simulink model "Feeder_1"  (Simulink 8.8)
settings: Solver=ode4  StartTime=0.0  StopTime=inf  FixedStep=Ts  RelTol=1e-3  EnableMultiTasking=on
PreLoadFcn:
  | Ts=125e-6;Core_Num = 0; np=1; nq=1; Vmin=.9;
PostLoadFcn:
  | Ts=125e-6;Core_Num = 0; np=1; nq=1; Vmin=.9;
InitFcn:
  | Ts=125e-6;Core_Num = 0; np=1; nq=1; Vmin=.9;
undefined symbols (not defined in the file or in its folder): another_event_name, DiscIntNeverNeededParam, I, j, Left, my_event_name, Right, type, V, X
libraries: powerlib x316, powerlib_meascontrol x227, simulink_extras x78, simulink x25, rtio_generic_c37_118 x22, ssn_lib x9, rtlab x6, powerlib_extras x3, artemis x1, rtio_opalrt_ml605ex1 x1, rtio_spectracom x1, rtio_generic_ethernet x1
(part 12 of 14)

== system Feeder_1/SM_NG/Single-Phase Dynamic Load48/model/PLL/adaptive filter ==
  u : Inport
  freq (Hz) : Inport  Port=2
  Gain : Gain  Gain=2*pi*2*0.707*2
  Gain1 : Gain  Gain=2*pi*2
  Product1 : Product  Inputs=***  RndMeth=Zero
  Product2 : Product  Inputs=**  RndMeth=Zero
  Product3 : Product  Inputs=***  RndMeth=Zero
  Sum1 : Sum  Inputs=+--  SaturateOnIntegerOverflow=on  InputSameDT=on  OutDataTypeStr=Inherit: Same as first input
  integrator1 : Integrator
  integrator2 : Integrator
  y : Outport
  wires:
  Product1/1 -> Sum1/2
  u/1 -> Product3/3
  freq (Hz)/1 -> Gain/1, Gain1/1
  Gain1/1 -> Product1/3, Product1/2, Product3/2, Product3/1
  Product3/1 -> Sum1/1
  integrator1/1 -> Product1/1, y/1
  Gain/1 -> Product2/2
  Product2/1 -> Sum1/3
  Sum1/1 -> integrator2/1
  integrator2/1 -> Product2/1, integrator1/1

== system Feeder_1/SM_NG/Single-Phase Dynamic Load48/model/PLL/adaptive mean ==
  u : Inport
  freq (Hz) : Inport  Port=2
  Fcn : Fcn  Expr=u(1)+1e-6
  Math Function : Math  Operator=reciprocal  SaturateOnIntegerOverflow=on
  Product1 : Product  Inputs=**  RndMeth=Zero
  Sum : Sum  Inputs=+-  SaturateOnIntegerOverflow=on  InputSameDT=on  OutDataTypeStr=Inherit: Same as first input
  Variable Transport Delay : VariableTransportDelay  MaximumDelay=1/40  MaximumPoints=4096
  integrator : Integrator
  y : Outport
  wires:
  Product1/1 -> y/1
  u/1 -> integrator/1
  Sum/1 -> Product1/1
  integrator/1 -> Variable Transport Delay/1, Sum/1
  Variable Transport Delay/1 -> Sum/2
  Math Function/1 -> Variable Transport Delay/2
  freq (Hz)/1 -> Fcn/1
  Fcn/1 -> Math Function/1, Product1/2

== system Feeder_1/SM_NG/Single-Phase Dynamic Load49/model/PLL/adaptive filter ==
  u : Inport
  freq (Hz) : Inport  Port=2
  Gain : Gain  Gain=2*pi*2*0.707*2
  Gain1 : Gain  Gain=2*pi*2
  Product1 : Product  Inputs=***  RndMeth=Zero
  Product2 : Product  Inputs=**  RndMeth=Zero
  Product3 : Product  Inputs=***  RndMeth=Zero
  Sum1 : Sum  Inputs=+--  SaturateOnIntegerOverflow=on  InputSameDT=on  OutDataTypeStr=Inherit: Same as first input
  integrator1 : Integrator
  integrator2 : Integrator
  y : Outport
  wires:
  Product1/1 -> Sum1/2
  u/1 -> Product3/3
  freq (Hz)/1 -> Gain/1, Gain1/1
  Gain1/1 -> Product1/3, Product1/2, Product3/2, Product3/1
  Product3/1 -> Sum1/1
  integrator1/1 -> Product1/1, y/1
  Gain/1 -> Product2/2
  Product2/1 -> Sum1/3
  Sum1/1 -> integrator2/1
  integrator2/1 -> Product2/1, integrator1/1

== system Feeder_1/SM_NG/Single-Phase Dynamic Load49/model/PLL/adaptive mean ==
  u : Inport
  freq (Hz) : Inport  Port=2
  Fcn : Fcn  Expr=u(1)+1e-6
  Math Function : Math  Operator=reciprocal  SaturateOnIntegerOverflow=on
  Product1 : Product  Inputs=**  RndMeth=Zero
  Sum : Sum  Inputs=+-  SaturateOnIntegerOverflow=on  InputSameDT=on  OutDataTypeStr=Inherit: Same as first input
  Variable Transport Delay : VariableTransportDelay  MaximumDelay=1/40  MaximumPoints=4096
  integrator : Integrator
  y : Outport
  wires:
  Product1/1 -> y/1
  u/1 -> integrator/1
  Sum/1 -> Product1/1
  integrator/1 -> Variable Transport Delay/1, Sum/1
  Variable Transport Delay/1 -> Sum/2
  Math Function/1 -> Variable Transport Delay/2
  freq (Hz)/1 -> Fcn/1
  Fcn/1 -> Math Function/1, Product1/2

== system Feeder_1/SM_NG/Single-Phase Dynamic Load50/model/PLL/adaptive filter ==
  u : Inport
  freq (Hz) : Inport  Port=2
  Gain : Gain  Gain=2*pi*2*0.707*2
  Gain1 : Gain  Gain=2*pi*2
  Product1 : Product  Inputs=***  RndMeth=Zero
  Product2 : Product  Inputs=**  RndMeth=Zero
  Product3 : Product  Inputs=***  RndMeth=Zero
  Sum1 : Sum  Inputs=+--  SaturateOnIntegerOverflow=on  InputSameDT=on  OutDataTypeStr=Inherit: Same as first input
  integrator1 : Integrator
  integrator2 : Integrator
  y : Outport
  wires:
  Product1/1 -> Sum1/2
  u/1 -> Product3/3
  freq (Hz)/1 -> Gain/1, Gain1/1
  Gain1/1 -> Product1/3, Product1/2, Product3/2, Product3/1
  Product3/1 -> Sum1/1
  integrator1/1 -> Product1/1, y/1
  Gain/1 -> Product2/2
  Product2/1 -> Sum1/3
  Sum1/1 -> integrator2/1
  integrator2/1 -> Product2/1, integrator1/1

== system Feeder_1/SM_NG/Single-Phase Dynamic Load50/model/PLL/adaptive mean ==
  u : Inport
  freq (Hz) : Inport  Port=2
  Fcn : Fcn  Expr=u(1)+1e-6
  Math Function : Math  Operator=reciprocal  SaturateOnIntegerOverflow=on
  Product1 : Product  Inputs=**  RndMeth=Zero
  Sum : Sum  Inputs=+-  SaturateOnIntegerOverflow=on  InputSameDT=on  OutDataTypeStr=Inherit: Same as first input
  Variable Transport Delay : VariableTransportDelay  MaximumDelay=1/40  MaximumPoints=4096
  integrator : Integrator
  y : Outport
  wires:
  Product1/1 -> y/1
  u/1 -> integrator/1
  Sum/1 -> Product1/1
  integrator/1 -> Variable Transport Delay/1, Sum/1
  Variable Transport Delay/1 -> Sum/2
  Math Function/1 -> Variable Transport Delay/2
  freq (Hz)/1 -> Fcn/1
  Fcn/1 -> Math Function/1, Product1/2

== system Feeder_1/SM_NG/Single-Phase Dynamic Load51/model/PLL/adaptive filter ==
  u : Inport
  freq (Hz) : Inport  Port=2
  Gain : Gain  Gain=2*pi*2*0.707*2
  Gain1 : Gain  Gain=2*pi*2
  Product1 : Product  Inputs=***  RndMeth=Zero
  Product2 : Product  Inputs=**  RndMeth=Zero
  Product3 : Product  Inputs=***  RndMeth=Zero
  Sum1 : Sum  Inputs=+--  SaturateOnIntegerOverflow=on  InputSameDT=on  OutDataTypeStr=Inherit: Same as first input
  integrator1 : Integrator
  integrator2 : Integrator
  y : Outport
  wires:
  Product1/1 -> Sum1/2
  u/1 -> Product3/3
  freq (Hz)/1 -> Gain/1, Gain1/1
  Gain1/1 -> Product1/3, Product1/2, Product3/2, Product3/1
  Product3/1 -> Sum1/1
  integrator1/1 -> Product1/1, y/1
  Gain/1 -> Product2/2
  Product2/1 -> Sum1/3
  Sum1/1 -> integrator2/1
  integrator2/1 -> Product2/1, integrator1/1

== system Feeder_1/SM_NG/Single-Phase Dynamic Load51/model/PLL/adaptive mean ==
  u : Inport
  freq (Hz) : Inport  Port=2
  Fcn : Fcn  Expr=u(1)+1e-6
  Math Function : Math  Operator=reciprocal  SaturateOnIntegerOverflow=on
  Product1 : Product  Inputs=**  RndMeth=Zero
  Sum : Sum  Inputs=+-  SaturateOnIntegerOverflow=on  InputSameDT=on  OutDataTypeStr=Inherit: Same as first input
  Variable Transport Delay : VariableTransportDelay  MaximumDelay=1/40  MaximumPoints=4096
  integrator : Integrator
  y : Outport
  wires:
  Product1/1 -> y/1
  u/1 -> integrator/1
  Sum/1 -> Product1/1
  integrator/1 -> Variable Transport Delay/1, Sum/1
  Variable Transport Delay/1 -> Sum/2
  Math Function/1 -> Variable Transport Delay/2
  freq (Hz)/1 -> Fcn/1
  Fcn/1 -> Math Function/1, Product1/2

== system Feeder_1/SM_NG/Single-Phase Dynamic Load52/model/PLL/adaptive filter ==
  u : Inport
  freq (Hz) : Inport  Port=2
  Gain : Gain  Gain=2*pi*2*0.707*2
  Gain1 : Gain  Gain=2*pi*2
  Product1 : Product  Inputs=***  RndMeth=Zero
  Product2 : Product  Inputs=**  RndMeth=Zero
  Product3 : Product  Inputs=***  RndMeth=Zero
  Sum1 : Sum  Inputs=+--  SaturateOnIntegerOverflow=on  InputSameDT=on  OutDataTypeStr=Inherit: Same as first input
  integrator1 : Integrator
  integrator2 : Integrator
  y : Outport
  wires:
  Product1/1 -> Sum1/2
  u/1 -> Product3/3
  freq (Hz)/1 -> Gain/1, Gain1/1
  Gain1/1 -> Product1/3, Product1/2, Product3/2, Product3/1
  Product3/1 -> Sum1/1
  integrator1/1 -> Product1/1, y/1
  Gain/1 -> Product2/2
  Product2/1 -> Sum1/3
  Sum1/1 -> integrator2/1
  integrator2/1 -> Product2/1, integrator1/1

== system Feeder_1/SM_NG/Single-Phase Dynamic Load52/model/PLL/adaptive mean ==
  u : Inport
  freq (Hz) : Inport  Port=2
  Fcn : Fcn  Expr=u(1)+1e-6
  Math Function : Math  Operator=reciprocal  SaturateOnIntegerOverflow=on
  Product1 : Product  Inputs=**  RndMeth=Zero
  Sum : Sum  Inputs=+-  SaturateOnIntegerOverflow=on  InputSameDT=on  OutDataTypeStr=Inherit: Same as first input
  Variable Transport Delay : VariableTransportDelay  MaximumDelay=1/40  MaximumPoints=4096
  integrator : Integrator
  y : Outport
  wires:
  Product1/1 -> y/1
  u/1 -> integrator/1
  Sum/1 -> Product1/1
  integrator/1 -> Variable Transport Delay/1, Sum/1
  Variable Transport Delay/1 -> Sum/2
  Math Function/1 -> Variable Transport Delay/2
  freq (Hz)/1 -> Fcn/1
  Fcn/1 -> Math Function/1, Product1/2

== system Feeder_1/SM_NG/Single-Phase Dynamic Load53/model/PLL/adaptive filter ==
  u : Inport
  freq (Hz) : Inport  Port=2
  Gain : Gain  Gain=2*pi*2*0.707*2
  Gain1 : Gain  Gain=2*pi*2
  Product1 : Product  Inputs=***  RndMeth=Zero
  Product2 : Product  Inputs=**  RndMeth=Zero
  Product3 : Product  Inputs=***  RndMeth=Zero
  Sum1 : Sum  Inputs=+--  SaturateOnIntegerOverflow=on  InputSameDT=on  OutDataTypeStr=Inherit: Same as first input
  integrator1 : Integrator
  integrator2 : Integrator
  y : Outport
  wires:
  Product1/1 -> Sum1/2
  u/1 -> Product3/3
  freq (Hz)/1 -> Gain/1, Gain1/1
  Gain1/1 -> Product1/3, Product1/2, Product3/2, Product3/1
  Product3/1 -> Sum1/1
  integrator1/1 -> Product1/1, y/1
  Gain/1 -> Product2/2
  Product2/1 -> Sum1/3
  Sum1/1 -> integrator2/1
  integrator2/1 -> Product2/1, integrator1/1

== system Feeder_1/SM_NG/Single-Phase Dynamic Load53/model/PLL/adaptive mean ==
  u : Inport
  freq (Hz) : Inport  Port=2
  Fcn : Fcn  Expr=u(1)+1e-6
  Math Function : Math  Operator=reciprocal  SaturateOnIntegerOverflow=on
  Product1 : Product  Inputs=**  RndMeth=Zero
  Sum : Sum  Inputs=+-  SaturateOnIntegerOverflow=on  InputSameDT=on  OutDataTypeStr=Inherit: Same as first input
  Variable Transport Delay : VariableTransportDelay  MaximumDelay=1/40  MaximumPoints=4096
  integrator : Integrator
  y : Outport
  wires:
  Product1/1 -> y/1
  u/1 -> integrator/1
  Sum/1 -> Product1/1
  integrator/1 -> Variable Transport Delay/1, Sum/1
  Variable Transport Delay/1 -> Sum/2
  Math Function/1 -> Variable Transport Delay/2
  freq (Hz)/1 -> Fcn/1
  Fcn/1 -> Math Function/1, Product1/2

== system Feeder_1/SM_NG/Single-Phase Dynamic Load54/model/PLL/adaptive filter ==
  u : Inport
  freq (Hz) : Inport  Port=2
  Gain : Gain  Gain=2*pi*2*0.707*2
  Gain1 : Gain  Gain=2*pi*2
  Product1 : Product  Inputs=***  RndMeth=Zero
  Product2 : Product  Inputs=**  RndMeth=Zero
  Product3 : Product  Inputs=***  RndMeth=Zero
  Sum1 : Sum  Inputs=+--  SaturateOnIntegerOverflow=on  InputSameDT=on  OutDataTypeStr=Inherit: Same as first input
  integrator1 : Integrator
  integrator2 : Integrator
  y : Outport
  wires:
  Product1/1 -> Sum1/2
  u/1 -> Product3/3
  freq (Hz)/1 -> Gain/1, Gain1/1
  Gain1/1 -> Product1/3, Product1/2, Product3/2, Product3/1
  Product3/1 -> Sum1/1
  integrator1/1 -> Product1/1, y/1
  Gain/1 -> Product2/2
  Product2/1 -> Sum1/3
  Sum1/1 -> integrator2/1
  integrator2/1 -> Product2/1, integrator1/1

== system Feeder_1/SM_NG/Single-Phase Dynamic Load54/model/PLL/adaptive mean ==
  u : Inport
  freq (Hz) : Inport  Port=2
  Fcn : Fcn  Expr=u(1)+1e-6
  Math Function : Math  Operator=reciprocal  SaturateOnIntegerOverflow=on
  Product1 : Product  Inputs=**  RndMeth=Zero
  Sum : Sum  Inputs=+-  SaturateOnIntegerOverflow=on  InputSameDT=on  OutDataTypeStr=Inherit: Same as first input
  Variable Transport Delay : VariableTransportDelay  MaximumDelay=1/40  MaximumPoints=4096
  integrator : Integrator
  y : Outport
  wires:
  Product1/1 -> y/1
  u/1 -> integrator/1
  Sum/1 -> Product1/1
  integrator/1 -> Variable Transport Delay/1, Sum/1
  Variable Transport Delay/1 -> Sum/2
  Math Function/1 -> Variable Transport Delay/2
  freq (Hz)/1 -> Fcn/1
  Fcn/1 -> Math Function/1, Product1/2

== system Feeder_1/SM_NG/Single-Phase Dynamic Load55/model/PLL/adaptive filter ==
  u : Inport
  freq (Hz) : Inport  Port=2
  Gain : Gain  Gain=2*pi*2*0.707*2
  Gain1 : Gain  Gain=2*pi*2
  Product1 : Product  Inputs=***  RndMeth=Zero
  Product2 : Product  Inputs=**  RndMeth=Zero
  Product3 : Product  Inputs=***  RndMeth=Zero
  Sum1 : Sum  Inputs=+--  SaturateOnIntegerOverflow=on  InputSameDT=on  OutDataTypeStr=Inherit: Same as first input
  integrator1 : Integrator
  integrator2 : Integrator
  y : Outport
  wires:
  Product1/1 -> Sum1/2
  u/1 -> Product3/3
  freq (Hz)/1 -> Gain/1, Gain1/1
  Gain1/1 -> Product1/3, Product1/2, Product3/2, Product3/1
  Product3/1 -> Sum1/1
  integrator1/1 -> Product1/1, y/1
  Gain/1 -> Product2/2
  Product2/1 -> Sum1/3
  Sum1/1 -> integrator2/1
  integrator2/1 -> Product2/1, integrator1/1

== system Feeder_1/SM_NG/Single-Phase Dynamic Load55/model/PLL/adaptive mean ==
  u : Inport
  freq (Hz) : Inport  Port=2
  Fcn : Fcn  Expr=u(1)+1e-6
  Math Function : Math  Operator=reciprocal  SaturateOnIntegerOverflow=on
  Product1 : Product  Inputs=**  RndMeth=Zero
  Sum : Sum  Inputs=+-  SaturateOnIntegerOverflow=on  InputSameDT=on  OutDataTypeStr=Inherit: Same as first input
  Variable Transport Delay : VariableTransportDelay  MaximumDelay=1/40  MaximumPoints=4096
  integrator : Integrator
  y : Outport
  wires:
  Product1/1 -> y/1
  u/1 -> integrator/1
  Sum/1 -> Product1/1
  integrator/1 -> Variable Transport Delay/1, Sum/1
  Variable Transport Delay/1 -> Sum/2
  Math Function/1 -> Variable Transport Delay/2
  freq (Hz)/1 -> Fcn/1
  Fcn/1 -> Math Function/1, Product1/2

== system Feeder_1/SM_NG/Single-Phase Dynamic Load56/model/PLL/adaptive filter ==
  u : Inport
  freq (Hz) : Inport  Port=2
  Gain : Gain  Gain=2*pi*2*0.707*2
  Gain1 : Gain  Gain=2*pi*2
  Product1 : Product  Inputs=***  RndMeth=Zero
  Product2 : Product  Inputs=**  RndMeth=Zero
  Product3 : Product  Inputs=***  RndMeth=Zero
  Sum1 : Sum  Inputs=+--  SaturateOnIntegerOverflow=on  InputSameDT=on  OutDataTypeStr=Inherit: Same as first input
  integrator1 : Integrator
  integrator2 : Integrator
  y : Outport
  wires:
  Product1/1 -> Sum1/2
  u/1 -> Product3/3
  freq (Hz)/1 -> Gain/1, Gain1/1
  Gain1/1 -> Product1/3, Product1/2, Product3/2, Product3/1
  Product3/1 -> Sum1/1
  integrator1/1 -> Product1/1, y/1
  Gain/1 -> Product2/2
  Product2/1 -> Sum1/3
  Sum1/1 -> integrator2/1
  integrator2/1 -> Product2/1, integrator1/1

== system Feeder_1/SM_NG/Single-Phase Dynamic Load56/model/PLL/adaptive mean ==
  u : Inport
  freq (Hz) : Inport  Port=2
  Fcn : Fcn  Expr=u(1)+1e-6
  Math Function : Math  Operator=reciprocal  SaturateOnIntegerOverflow=on
  Product1 : Product  Inputs=**  RndMeth=Zero
  Sum : Sum  Inputs=+-  SaturateOnIntegerOverflow=on  InputSameDT=on  OutDataTypeStr=Inherit: Same as first input
  Variable Transport Delay : VariableTransportDelay  MaximumDelay=1/40  MaximumPoints=4096
  integrator : Integrator
  y : Outport
  wires:
  Product1/1 -> y/1
  u/1 -> integrator/1
  Sum/1 -> Product1/1
  integrator/1 -> Variable Transport Delay/1, Sum/1
  Variable Transport Delay/1 -> Sum/2
  Math Function/1 -> Variable Transport Delay/2
  freq (Hz)/1 -> Fcn/1
  Fcn/1 -> Math Function/1, Product1/2

== system Feeder_1/SM_NG/Single-Phase Dynamic Load57/model/PLL/adaptive filter ==
  u : Inport
  freq (Hz) : Inport  Port=2
  Gain : Gain  Gain=2*pi*2*0.707*2
  Gain1 : Gain  Gain=2*pi*2
  Product1 : Product  Inputs=***  RndMeth=Zero
  Product2 : Product  Inputs=**  RndMeth=Zero
  Product3 : Product  Inputs=***  RndMeth=Zero
  Sum1 : Sum  Inputs=+--  SaturateOnIntegerOverflow=on  InputSameDT=on  OutDataTypeStr=Inherit: Same as first input
  integrator1 : Integrator
  integrator2 : Integrator
  y : Outport
  wires:
  Product1/1 -> Sum1/2
  u/1 -> Product3/3
  freq (Hz)/1 -> Gain/1, Gain1/1
  Gain1/1 -> Product1/3, Product1/2, Product3/2, Product3/1
  Product3/1 -> Sum1/1
  integrator1/1 -> Product1/1, y/1
  Gain/1 -> Product2/2
  Product2/1 -> Sum1/3
  Sum1/1 -> integrator2/1
  integrator2/1 -> Product2/1, integrator1/1

== system Feeder_1/SM_NG/Single-Phase Dynamic Load57/model/PLL/adaptive mean ==
  u : Inport
  freq (Hz) : Inport  Port=2
  Fcn : Fcn  Expr=u(1)+1e-6
  Math Function : Math  Operator=reciprocal  SaturateOnIntegerOverflow=on
  Product1 : Product  Inputs=**  RndMeth=Zero
  Sum : Sum  Inputs=+-  SaturateOnIntegerOverflow=on  InputSameDT=on  OutDataTypeStr=Inherit: Same as first input
  Variable Transport Delay : VariableTransportDelay  MaximumDelay=1/40  MaximumPoints=4096
  integrator : Integrator
  y : Outport
  wires:
  Product1/1 -> y/1
  u/1 -> integrator/1
  Sum/1 -> Product1/1
  integrator/1 -> Variable Transport Delay/1, Sum/1
  Variable Transport Delay/1 -> Sum/2
  Math Function/1 -> Variable Transport Delay/2
  freq (Hz)/1 -> Fcn/1
  Fcn/1 -> Math Function/1, Product1/2

== system Feeder_1/SM_NG/Single-Phase Dynamic Load58/model/PLL/adaptive filter ==
  u : Inport
  freq (Hz) : Inport  Port=2
  Gain : Gain  Gain=2*pi*2*0.707*2
  Gain1 : Gain  Gain=2*pi*2
  Product1 : Product  Inputs=***  RndMeth=Zero
  Product2 : Product  Inputs=**  RndMeth=Zero
  Product3 : Product  Inputs=***  RndMeth=Zero
  Sum1 : Sum  Inputs=+--  SaturateOnIntegerOverflow=on  InputSameDT=on  OutDataTypeStr=Inherit: Same as first input
  integrator1 : Integrator
  integrator2 : Integrator
  y : Outport
  wires:
  Product1/1 -> Sum1/2
  u/1 -> Product3/3
  freq (Hz)/1 -> Gain/1, Gain1/1
  Gain1/1 -> Product1/3, Product1/2, Product3/2, Product3/1
  Product3/1 -> Sum1/1
  integrator1/1 -> Product1/1, y/1
  Gain/1 -> Product2/2
  Product2/1 -> Sum1/3
  Sum1/1 -> integrator2/1
  integrator2/1 -> Product2/1, integrator1/1

== system Feeder_1/SM_NG/Single-Phase Dynamic Load58/model/PLL/adaptive mean ==
  u : Inport
  freq (Hz) : Inport  Port=2
  Fcn : Fcn  Expr=u(1)+1e-6
  Math Function : Math  Operator=reciprocal  SaturateOnIntegerOverflow=on
  Product1 : Product  Inputs=**  RndMeth=Zero
  Sum : Sum  Inputs=+-  SaturateOnIntegerOverflow=on  InputSameDT=on  OutDataTypeStr=Inherit: Same as first input
  Variable Transport Delay : VariableTransportDelay  MaximumDelay=1/40  MaximumPoints=4096
  integrator : Integrator
  y : Outport
  wires:
  Product1/1 -> y/1
  u/1 -> integrator/1
  Sum/1 -> Product1/1
  integrator/1 -> Variable Transport Delay/1, Sum/1
  Variable Transport Delay/1 -> Sum/2
  Math Function/1 -> Variable Transport Delay/2
  freq (Hz)/1 -> Fcn/1
  Fcn/1 -> Math Function/1, Product1/2

== system Feeder_1/SM_NG/Single-Phase Dynamic Load59/model/PLL/adaptive filter ==
  u : Inport
  freq (Hz) : Inport  Port=2
  Gain : Gain  Gain=2*pi*2*0.707*2
  Gain1 : Gain  Gain=2*pi*2
  Product1 : Product  Inputs=***  RndMeth=Zero
  Product2 : Product  Inputs=**  RndMeth=Zero
  Product3 : Product  Inputs=***  RndMeth=Zero
  Sum1 : Sum  Inputs=+--  SaturateOnIntegerOverflow=on  InputSameDT=on  OutDataTypeStr=Inherit: Same as first input
  integrator1 : Integrator
  integrator2 : Integrator
  y : Outport
  wires:
  Product1/1 -> Sum1/2
  u/1 -> Product3/3
  freq (Hz)/1 -> Gain/1, Gain1/1
  Gain1/1 -> Product1/3, Product1/2, Product3/2, Product3/1
  Product3/1 -> Sum1/1
  integrator1/1 -> Product1/1, y/1
  Gain/1 -> Product2/2
  Product2/1 -> Sum1/3
  Sum1/1 -> integrator2/1
  integrator2/1 -> Product2/1, integrator1/1

== system Feeder_1/SM_NG/Single-Phase Dynamic Load59/model/PLL/adaptive mean ==
  u : Inport
  freq (Hz) : Inport  Port=2
  Fcn : Fcn  Expr=u(1)+1e-6
  Math Function : Math  Operator=reciprocal  SaturateOnIntegerOverflow=on
  Product1 : Product  Inputs=**  RndMeth=Zero
  Sum : Sum  Inputs=+-  SaturateOnIntegerOverflow=on  InputSameDT=on  OutDataTypeStr=Inherit: Same as first input
  Variable Transport Delay : VariableTransportDelay  MaximumDelay=1/40  MaximumPoints=4096
  integrator : Integrator
  y : Outport
  wires:
  Product1/1 -> y/1
  u/1 -> integrator/1
  Sum/1 -> Product1/1
  integrator/1 -> Variable Transport Delay/1, Sum/1
  Variable Transport Delay/1 -> Sum/2
  Math Function/1 -> Variable Transport Delay/2
  freq (Hz)/1 -> Fcn/1
  Fcn/1 -> Math Function/1, Product1/2

== system Feeder_1/SM_NG/Single-Phase Dynamic Load60/model/PLL/adaptive filter ==
  u : Inport
  freq (Hz) : Inport  Port=2
  Gain : Gain  Gain=2*pi*2*0.707*2
  Gain1 : Gain  Gain=2*pi*2
  Product1 : Product  Inputs=***  RndMeth=Zero
  Product2 : Product  Inputs=**  RndMeth=Zero
  Product3 : Product  Inputs=***  RndMeth=Zero
  Sum1 : Sum  Inputs=+--  SaturateOnIntegerOverflow=on  InputSameDT=on  OutDataTypeStr=Inherit: Same as first input
  integrator1 : Integrator
  integrator2 : Integrator
  y : Outport
  wires:
  Product1/1 -> Sum1/2
  u/1 -> Product3/3
  freq (Hz)/1 -> Gain/1, Gain1/1
  Gain1/1 -> Product1/3, Product1/2, Product3/2, Product3/1
  Product3/1 -> Sum1/1
  integrator1/1 -> Product1/1, y/1
  Gain/1 -> Product2/2
  Product2/1 -> Sum1/3
  Sum1/1 -> integrator2/1
  integrator2/1 -> Product2/1, integrator1/1

== system Feeder_1/SM_NG/Single-Phase Dynamic Load60/model/PLL/adaptive mean ==
  u : Inport
  freq (Hz) : Inport  Port=2
  Fcn : Fcn  Expr=u(1)+1e-6
  Math Function : Math  Operator=reciprocal  SaturateOnIntegerOverflow=on
  Product1 : Product  Inputs=**  RndMeth=Zero
  Sum : Sum  Inputs=+-  SaturateOnIntegerOverflow=on  InputSameDT=on  OutDataTypeStr=Inherit: Same as first input
  Variable Transport Delay : VariableTransportDelay  MaximumDelay=1/40  MaximumPoints=4096
  integrator : Integrator
  y : Outport
  wires:
  Product1/1 -> y/1
  u/1 -> integrator/1
  Sum/1 -> Product1/1
  integrator/1 -> Variable Transport Delay/1, Sum/1
  Variable Transport Delay/1 -> Sum/2
  Math Function/1 -> Variable Transport Delay/2
  freq (Hz)/1 -> Fcn/1
  Fcn/1 -> Math Function/1, Product1/2

== system Feeder_1/SM_NG/Subsystem/Single-Phase Voltage Regulator1/SSN OLTC xfo v2/DC source_a ==
  I1A_V : powerlib/Electrical Sources/DC Voltage Source  Amplitude=0  Measurements=None
  Conn1 : PMIOPort  Port=1  Side=Left
  Conn2 : PMIOPort  Port=2  Side=Right
  connections:
  Conn1/RConn1 -- I1A_V/LConn1
  Conn2/RConn1 -- I1A_V/RConn1

== system Feeder_1/SM_NG/Subsystem/Single-Phase Voltage Regulator1/SSN OLTC xfo v2/DC source_b ==
  I1B_V : powerlib/Electrical Sources/DC Voltage Source  Amplitude=0  Measurements=None
  Conn3 : PMIOPort  Port=1  Side=Left
  Conn4 : PMIOPort  Port=2  Side=Right
  connections:
  Conn4/RConn1 -- I1B_V/RConn1
  Conn3/RConn1 -- I1B_V/LConn1

== system Feeder_1/SM_NG/Subsystem/Single-Phase Voltage Regulator1/SSN OLTC xfo v2/DC source_c ==
  I1C_V : powerlib/Electrical Sources/DC Voltage Source  Amplitude=0  Measurements=None
  Conn1 : PMIOPort  Port=1  Side=Left
  Conn2 : PMIOPort  Port=2  Side=Right
  connections:
  Conn2/RConn1 -- I1C_V/RConn1
  Conn1/RConn1 -- I1C_V/LConn1

== system Feeder_1/SM_NG/Subsystem/Single-Phase Voltage Regulator1/SSN OLTC xfo v2/DC source_d ==
  I1D_V : powerlib/Electrical Sources/DC Voltage Source  Amplitude=0  Measurements=None
  Conn3 : PMIOPort  Port=1  Side=Left
  Conn4 : PMIOPort  Port=2  Side=Right
  connections:
  Conn3/RConn1 -- I1D_V/LConn1
  Conn4/RConn1 -- I1D_V/RConn1

== system Feeder_1/SM_NG/Subsystem/Single-Phase Voltage Regulator1/SSN OLTC xfo v2/SSS-SM equations ==
  A : Inport
  B : Inport  Port=2
  C : Inport  Port=3
  u : Inport  Port=4
  Flux0 : Inport  Port=5
  Bphic : Inport  Port=6
  be : Inport  Port=7
  Constant : Constant
  Discretize : Subsystem
  Product{1..3,5..6} (5 alike) : Product  Multiplication=Matrix(*)  SaturateOnIntegerOverflow=on  OutDataTypeStr=Inherit: Same as first input
  Sum1 : Sum  Inputs=-+  SaturateOnIntegerOverflow=on
  Sum2 : Sum  Inputs=+++  SaturateOnIntegerOverflow=on
  Sum3 : Sum  SaturateOnIntegerOverflow=on
  mult1 : Product
  u5 : Constant  Value=eye(3,3)
  z-1 : UnitDelay  SampleTime=Ts
  Y : Outport
  Ihist : Outport  Port=2
  x : Outport  Port=3
  wires:
  u5/1 -> Discretize/3(Unity)
  Product2/1 -> Y/1
  A/1 -> Discretize/1(Ac)
  B/1 -> Discretize/2(Bc)
  C/1 -> Product2/1, Product6/1
  Product6/1 -> Ihist/1
  Product5/1 -> Sum3/2, mult1/1
  Product3/1 -> Sum2/1
  Sum3/1 -> Product3/2, x/1  "new_x"
  Sum2/1 -> z-1/1, Product6/2
  Discretize/1(Ad) -> Product3/1
  u/1 -> Product5/2
  z-1/1 -> Sum3/1
  Discretize/2(Bd) -> Product5/1, Product2/2
  Discretize/3(Bdin) -> Product1/1
  Product1/1 -> Sum2/3
  Flux0/1 -> Product1/2
  Bphic/1 -> Discretize/4(Bphic)
  Constant/1 -> Sum1/2
  mult1/1 -> Sum2/2
  Sum1/1 -> mult1/2  "=1 if trapeze           =0 if BE"
  be/1 -> Discretize/5(be), Sum1/1

== system Feeder_1/SM_NG/Subsystem/Single-Phase Voltage Regulator1/SSN OLTC xfo v2/Update Matrix L ==
  k : Inport
  L2 : Inport  Port=2
  Lin : Inport  Port=3
  "L2->(2,2) " : Assignment  NumberOfDimensions=2  IndexOptions=Index vector (dialog),Index vector (dialog)  Indices=[2],[2]  OutputSizes=1,1
  k->(2,3) : Assignment  NumberOfDimensions=2  IndexOptions=Index vector (dialog),Index vector (dialog)  Indices=[2],[3]  OutputSizes=1,1
  L : Outport
  wires:
  "L2->(2,2) "/1 -> L/1
  L2/1 -> "L2->(2,2) "/2
  Lin/1 -> k->(2,3)/1
  k/1 -> k->(2,3)/2
  k->(2,3)/1 -> "L2->(2,2) "/1

== system Feeder_1/SM_NG/Subsystem/Single-Phase Voltage Regulator1/SSN OLTC xfo v2/Update Matrix R ==
  R2 : Inport
  Rin : Inport  Port=2
  k : Inport  Port=3
  Rcore : Inport  Port=4
  Rcore/Lcore : Inport  Port=5
  "-R2->(2,2) " : Assignment  NumberOfDimensions=2  IndexOptions=Index vector (dialog),Index vector (dialog)  Indices=[2],[2]  OutputSizes=1,1
  -Rm/Lm->(3,3) : Assignment  NumberOfDimensions=2  IndexOptions=Index vector (dialog),Index vector (dialog)  Indices=3,3  OutputSizes=1,1
  Gain : Gain  Gain=-1
  Gain1 : Gain  Gain=-1
  Product1 : Product  RndMeth=Zero
  kRm->(3,2) : Assignment  NumberOfDimensions=2  IndexOptions=Index vector (dialog),Index vector (dialog)  Indices=3,2  OutputSizes=1,1
  R : Outport
  wires:
  "-R2->(2,2) "/1 -> kRm->(3,2)/1
  R2/1 -> Gain/1
  Rin/1 -> "-R2->(2,2) "/1
  Gain/1 -> "-R2->(2,2) "/2
  k/1 -> Product1/2
  Product1/1 -> kRm->(3,2)/2
  kRm->(3,2)/1 -> -Rm/Lm->(3,3)/1
  -Rm/Lm->(3,3)/1 -> R/1
  Rcore/1 -> Product1/1
  Gain1/1 -> -Rm/Lm->(3,3)/2
  Rcore/Lcore/1 -> Gain1/1

== system Feeder_1/SM_NG/Subsystem/Single-Phase Voltage Regulator1/SSN OLTC xfo v2/conn_down_c ==
  b2 : PMIOPort  Port=1  Side=Right
  b1 : PMIOPort  Port=2  Side=Left
  connections:
  b1/RConn1 -- b2/RConn1

== system Feeder_1/SM_NG/Subsystem/Single-Phase Voltage Regulator1/SSN OLTC xfo v2/conn_down_d ==
  b2 : PMIOPort  Port=1  Side=Right
  b1 : PMIOPort  Port=2  Side=Left
  connections:
  b1/RConn1 -- b2/RConn1

== system Feeder_1/SM_NG/Subsystem/Single-Phase Voltage Regulator1/SSN OLTC xfo v2/conn_up_c ==
  b2 : PMIOPort  Port=1  Side=Right
  b1 : PMIOPort  Port=2  Side=Left
  connections:
  b1/RConn1 -- b2/RConn1

== system Feeder_1/SM_NG/Subsystem/Single-Phase Voltage Regulator1/SSN OLTC xfo v2/conn_up_d ==
  b2 : PMIOPort  Port=1  Side=Right
  b1 : PMIOPort  Port=2  Side=Left
  connections:
  b1/RConn1 -- b2/RConn1

== system Feeder_1/SM_NG/Subsystem/Single-Phase Voltage Regulator2/SSN OLTC xfo v2/DC source_a ==
  I1A_V : powerlib/Electrical Sources/DC Voltage Source  Amplitude=0  Measurements=None
  Conn1 : PMIOPort  Port=1  Side=Left
  Conn2 : PMIOPort  Port=2  Side=Right
  connections:
  Conn1/RConn1 -- I1A_V/LConn1
  Conn2/RConn1 -- I1A_V/RConn1

== system Feeder_1/SM_NG/Subsystem/Single-Phase Voltage Regulator2/SSN OLTC xfo v2/DC source_b ==
  I1B_V : powerlib/Electrical Sources/DC Voltage Source  Amplitude=0  Measurements=None
  Conn3 : PMIOPort  Port=1  Side=Left
  Conn4 : PMIOPort  Port=2  Side=Right
  connections:
  Conn4/RConn1 -- I1B_V/RConn1
  Conn3/RConn1 -- I1B_V/LConn1

== system Feeder_1/SM_NG/Subsystem/Single-Phase Voltage Regulator2/SSN OLTC xfo v2/DC source_c ==
  I1C_V : powerlib/Electrical Sources/DC Voltage Source  Amplitude=0  Measurements=None
  Conn1 : PMIOPort  Port=1  Side=Left
  Conn2 : PMIOPort  Port=2  Side=Right
  connections:
  Conn2/RConn1 -- I1C_V/RConn1
  Conn1/RConn1 -- I1C_V/LConn1

== system Feeder_1/SM_NG/Subsystem/Single-Phase Voltage Regulator2/SSN OLTC xfo v2/DC source_d ==
  I1D_V : powerlib/Electrical Sources/DC Voltage Source  Amplitude=0  Measurements=None
  Conn3 : PMIOPort  Port=1  Side=Left
  Conn4 : PMIOPort  Port=2  Side=Right
  connections:
  Conn3/RConn1 -- I1D_V/LConn1
  Conn4/RConn1 -- I1D_V/RConn1

== system Feeder_1/SM_NG/Subsystem/Single-Phase Voltage Regulator2/SSN OLTC xfo v2/SSS-SM equations ==
  A : Inport
  B : Inport  Port=2
  C : Inport  Port=3
  u : Inport  Port=4
  Flux0 : Inport  Port=5
  Bphic : Inport  Port=6
  be : Inport  Port=7
  Constant : Constant
  Discretize : Subsystem
  Product{1..3,5..6} (5 alike) : Product  Multiplication=Matrix(*)  SaturateOnIntegerOverflow=on  OutDataTypeStr=Inherit: Same as first input
  Sum1 : Sum  Inputs=-+  SaturateOnIntegerOverflow=on
  Sum2 : Sum  Inputs=+++  SaturateOnIntegerOverflow=on
  Sum3 : Sum  SaturateOnIntegerOverflow=on
  mult1 : Product
  u5 : Constant  Value=eye(3,3)
  z-1 : UnitDelay  SampleTime=Ts
  Y : Outport
  Ihist : Outport  Port=2
  x : Outport  Port=3
  wires:
  u5/1 -> Discretize/3(Unity)
  Product2/1 -> Y/1
  A/1 -> Discretize/1(Ac)
  B/1 -> Discretize/2(Bc)
  C/1 -> Product2/1, Product6/1
  Product6/1 -> Ihist/1
  Product5/1 -> Sum3/2, mult1/1
  Product3/1 -> Sum2/1
  Sum3/1 -> Product3/2, x/1  "new_x"
  Sum2/1 -> z-1/1, Product6/2
  Discretize/1(Ad) -> Product3/1
  u/1 -> Product5/2
  z-1/1 -> Sum3/1
  Discretize/2(Bd) -> Product5/1, Product2/2
  Discretize/3(Bdin) -> Product1/1
  Product1/1 -> Sum2/3
  Flux0/1 -> Product1/2
  Bphic/1 -> Discretize/4(Bphic)
  Constant/1 -> Sum1/2
  mult1/1 -> Sum2/2
  Sum1/1 -> mult1/2  "=1 if trapeze           =0 if BE"
  be/1 -> Discretize/5(be), Sum1/1

== system Feeder_1/SM_NG/Subsystem/Single-Phase Voltage Regulator2/SSN OLTC xfo v2/Update Matrix L ==
  k : Inport
  L2 : Inport  Port=2
  Lin : Inport  Port=3
  "L2->(2,2) " : Assignment  NumberOfDimensions=2  IndexOptions=Index vector (dialog),Index vector (dialog)  Indices=[2],[2]  OutputSizes=1,1
  k->(2,3) : Assignment  NumberOfDimensions=2  IndexOptions=Index vector (dialog),Index vector (dialog)  Indices=[2],[3]  OutputSizes=1,1
  L : Outport
  wires:
  "L2->(2,2) "/1 -> L/1
  L2/1 -> "L2->(2,2) "/2
  Lin/1 -> k->(2,3)/1
  k/1 -> k->(2,3)/2
  k->(2,3)/1 -> "L2->(2,2) "/1

== system Feeder_1/SM_NG/Subsystem/Single-Phase Voltage Regulator2/SSN OLTC xfo v2/Update Matrix R ==
  R2 : Inport
  Rin : Inport  Port=2
  k : Inport  Port=3
  Rcore : Inport  Port=4
  Rcore/Lcore : Inport  Port=5
  "-R2->(2,2) " : Assignment  NumberOfDimensions=2  IndexOptions=Index vector (dialog),Index vector (dialog)  Indices=[2],[2]  OutputSizes=1,1
  -Rm/Lm->(3,3) : Assignment  NumberOfDimensions=2  IndexOptions=Index vector (dialog),Index vector (dialog)  Indices=3,3  OutputSizes=1,1
  Gain : Gain  Gain=-1
  Gain1 : Gain  Gain=-1
  Product1 : Product  RndMeth=Zero
  kRm->(3,2) : Assignment  NumberOfDimensions=2  IndexOptions=Index vector (dialog),Index vector (dialog)  Indices=3,2  OutputSizes=1,1
  R : Outport
  wires:
  "-R2->(2,2) "/1 -> kRm->(3,2)/1
  R2/1 -> Gain/1
  Rin/1 -> "-R2->(2,2) "/1
  Gain/1 -> "-R2->(2,2) "/2
  k/1 -> Product1/2
  Product1/1 -> kRm->(3,2)/2
  kRm->(3,2)/1 -> -Rm/Lm->(3,3)/1
  -Rm/Lm->(3,3)/1 -> R/1
  Rcore/1 -> Product1/1
  Gain1/1 -> -Rm/Lm->(3,3)/2
  Rcore/Lcore/1 -> Gain1/1

== system Feeder_1/SM_NG/Subsystem/Single-Phase Voltage Regulator2/SSN OLTC xfo v2/conn_down_c ==
  b2 : PMIOPort  Port=1  Side=Right
  b1 : PMIOPort  Port=2  Side=Left
  connections:
  b1/RConn1 -- b2/RConn1

== system Feeder_1/SM_NG/Subsystem/Single-Phase Voltage Regulator2/SSN OLTC xfo v2/conn_down_d ==
  b2 : PMIOPort  Port=1  Side=Right
  b1 : PMIOPort  Port=2  Side=Left
  connections:
  b1/RConn1 -- b2/RConn1

== system Feeder_1/SM_NG/Subsystem/Single-Phase Voltage Regulator2/SSN OLTC xfo v2/conn_up_c ==
  b2 : PMIOPort  Port=1  Side=Right
  b1 : PMIOPort  Port=2  Side=Left
  connections:
  b1/RConn1 -- b2/RConn1

== system Feeder_1/SM_NG/Subsystem/Single-Phase Voltage Regulator2/SSN OLTC xfo v2/conn_up_d ==
  b2 : PMIOPort  Port=1  Side=Right
  b1 : PMIOPort  Port=2  Side=Left
  connections:
  b1/RConn1 -- b2/RConn1

== system Feeder_1/SM_NG/Subsystem/Single-Phase Voltage Regulator3/SSN OLTC xfo v2/DC source_a ==
  I1A_V : powerlib/Electrical Sources/DC Voltage Source  Amplitude=0  Measurements=None
  Conn1 : PMIOPort  Port=1  Side=Left
  Conn2 : PMIOPort  Port=2  Side=Right
  connections:
  Conn1/RConn1 -- I1A_V/LConn1
  Conn2/RConn1 -- I1A_V/RConn1

== system Feeder_1/SM_NG/Subsystem/Single-Phase Voltage Regulator3/SSN OLTC xfo v2/DC source_b ==
  I1B_V : powerlib/Electrical Sources/DC Voltage Source  Amplitude=0  Measurements=None
  Conn3 : PMIOPort  Port=1  Side=Left
  Conn4 : PMIOPort  Port=2  Side=Right
  connections:
  Conn4/RConn1 -- I1B_V/RConn1
  Conn3/RConn1 -- I1B_V/LConn1

== system Feeder_1/SM_NG/Subsystem/Single-Phase Voltage Regulator3/SSN OLTC xfo v2/DC source_c ==
  I1C_V : powerlib/Electrical Sources/DC Voltage Source  Amplitude=0  Measurements=None
  Conn1 : PMIOPort  Port=1  Side=Left
  Conn2 : PMIOPort  Port=2  Side=Right
  connections:
  Conn2/RConn1 -- I1C_V/RConn1
  Conn1/RConn1 -- I1C_V/LConn1

== system Feeder_1/SM_NG/Subsystem/Single-Phase Voltage Regulator3/SSN OLTC xfo v2/DC source_d ==
  I1D_V : powerlib/Electrical Sources/DC Voltage Source  Amplitude=0  Measurements=None
  Conn3 : PMIOPort  Port=1  Side=Left
  Conn4 : PMIOPort  Port=2  Side=Right
  connections:
  Conn3/RConn1 -- I1D_V/LConn1
  Conn4/RConn1 -- I1D_V/RConn1

== system Feeder_1/SM_NG/Subsystem/Single-Phase Voltage Regulator3/SSN OLTC xfo v2/SSS-SM equations ==
  A : Inport
  B : Inport  Port=2
  C : Inport  Port=3
  u : Inport  Port=4
  Flux0 : Inport  Port=5
  Bphic : Inport  Port=6
  be : Inport  Port=7
  Constant : Constant
  Discretize : Subsystem
  Product{1..3,5..6} (5 alike) : Product  Multiplication=Matrix(*)  SaturateOnIntegerOverflow=on  OutDataTypeStr=Inherit: Same as first input
  Sum1 : Sum  Inputs=-+  SaturateOnIntegerOverflow=on
  Sum2 : Sum  Inputs=+++  SaturateOnIntegerOverflow=on
  Sum3 : Sum  SaturateOnIntegerOverflow=on
  mult1 : Product
  u5 : Constant  Value=eye(3,3)
  z-1 : UnitDelay  SampleTime=Ts
  Y : Outport
  Ihist : Outport  Port=2
  x : Outport  Port=3
  wires:
  u5/1 -> Discretize/3(Unity)
  Product2/1 -> Y/1
  A/1 -> Discretize/1(Ac)
  B/1 -> Discretize/2(Bc)
  C/1 -> Product2/1, Product6/1
  Product6/1 -> Ihist/1
  Product5/1 -> Sum3/2, mult1/1
  Product3/1 -> Sum2/1
  Sum3/1 -> Product3/2, x/1  "new_x"
  Sum2/1 -> z-1/1, Product6/2
  Discretize/1(Ad) -> Product3/1
  u/1 -> Product5/2
  z-1/1 -> Sum3/1
  Discretize/2(Bd) -> Product5/1, Product2/2
  Discretize/3(Bdin) -> Product1/1
  Product1/1 -> Sum2/3
  Flux0/1 -> Product1/2
  Bphic/1 -> Discretize/4(Bphic)
  Constant/1 -> Sum1/2
  mult1/1 -> Sum2/2
  Sum1/1 -> mult1/2  "=1 if trapeze           =0 if BE"
  be/1 -> Discretize/5(be), Sum1/1

== system Feeder_1/SM_NG/Subsystem/Single-Phase Voltage Regulator3/SSN OLTC xfo v2/Update Matrix L ==
  k : Inport
  L2 : Inport  Port=2
  Lin : Inport  Port=3
  "L2->(2,2) " : Assignment  NumberOfDimensions=2  IndexOptions=Index vector (dialog),Index vector (dialog)  Indices=[2],[2]  OutputSizes=1,1
  k->(2,3) : Assignment  NumberOfDimensions=2  IndexOptions=Index vector (dialog),Index vector (dialog)  Indices=[2],[3]  OutputSizes=1,1
  L : Outport
  wires:
  "L2->(2,2) "/1 -> L/1
  L2/1 -> "L2->(2,2) "/2
  Lin/1 -> k->(2,3)/1
  k/1 -> k->(2,3)/2
  k->(2,3)/1 -> "L2->(2,2) "/1

== system Feeder_1/SM_NG/Subsystem/Single-Phase Voltage Regulator3/SSN OLTC xfo v2/Update Matrix R ==
  R2 : Inport
  Rin : Inport  Port=2
  k : Inport  Port=3
  Rcore : Inport  Port=4
  Rcore/Lcore : Inport  Port=5
  "-R2->(2,2) " : Assignment  NumberOfDimensions=2  IndexOptions=Index vector (dialog),Index vector (dialog)  Indices=[2],[2]  OutputSizes=1,1
  -Rm/Lm->(3,3) : Assignment  NumberOfDimensions=2  IndexOptions=Index vector (dialog),Index vector (dialog)  Indices=3,3  OutputSizes=1,1
  Gain : Gain  Gain=-1
  Gain1 : Gain  Gain=-1
  Product1 : Product  RndMeth=Zero
  kRm->(3,2) : Assignment  NumberOfDimensions=2  IndexOptions=Index vector (dialog),Index vector (dialog)  Indices=3,2  OutputSizes=1,1
  R : Outport
  wires:
  "-R2->(2,2) "/1 -> kRm->(3,2)/1
  R2/1 -> Gain/1
  Rin/1 -> "-R2->(2,2) "/1
  Gain/1 -> "-R2->(2,2) "/2
  k/1 -> Product1/2
  Product1/1 -> kRm->(3,2)/2
  kRm->(3,2)/1 -> -Rm/Lm->(3,3)/1
  -Rm/Lm->(3,3)/1 -> R/1
  Rcore/1 -> Product1/1
  Gain1/1 -> -Rm/Lm->(3,3)/2
  Rcore/Lcore/1 -> Gain1/1

== system Feeder_1/SM_NG/Subsystem/Single-Phase Voltage Regulator3/SSN OLTC xfo v2/conn_down_c ==
  b2 : PMIOPort  Port=1  Side=Right
  b1 : PMIOPort  Port=2  Side=Left
  connections:
  b1/RConn1 -- b2/RConn1

== system Feeder_1/SM_NG/Subsystem/Single-Phase Voltage Regulator3/SSN OLTC xfo v2/conn_down_d ==
  b2 : PMIOPort  Port=1  Side=Right
  b1 : PMIOPort  Port=2  Side=Left
  connections:
  b1/RConn1 -- b2/RConn1

== system Feeder_1/SM_NG/Subsystem/Single-Phase Voltage Regulator3/SSN OLTC xfo v2/conn_up_c ==
  b2 : PMIOPort  Port=1  Side=Right
  b1 : PMIOPort  Port=2  Side=Left
  connections:
  b1/RConn1 -- b2/RConn1

== system Feeder_1/SM_NG/Subsystem/Single-Phase Voltage Regulator3/SSN OLTC xfo v2/conn_up_d ==
  b2 : PMIOPort  Port=1  Side=Right
  b1 : PMIOPort  Port=2  Side=Left
  connections:
  b1/RConn1 -- b2/RConn1

== system Feeder_1/SS_PMU/Subsystem1/Subsystem/Subsystem1/Degree to radian1 ==
  Degree : Inport
  Constant : Constant  Value=pi
  Constant1 : Constant  Value=180
  Divide : Product  Inputs=*/
  Product : Product  RndMeth=Zero
  Radian : Outport
  wires:
  Divide/1 -> Radian/1
  Degree/1 -> Product/1
  Constant1/1 -> Divide/2
  Product/1 -> Divide/1
  Constant/1 -> Product/2

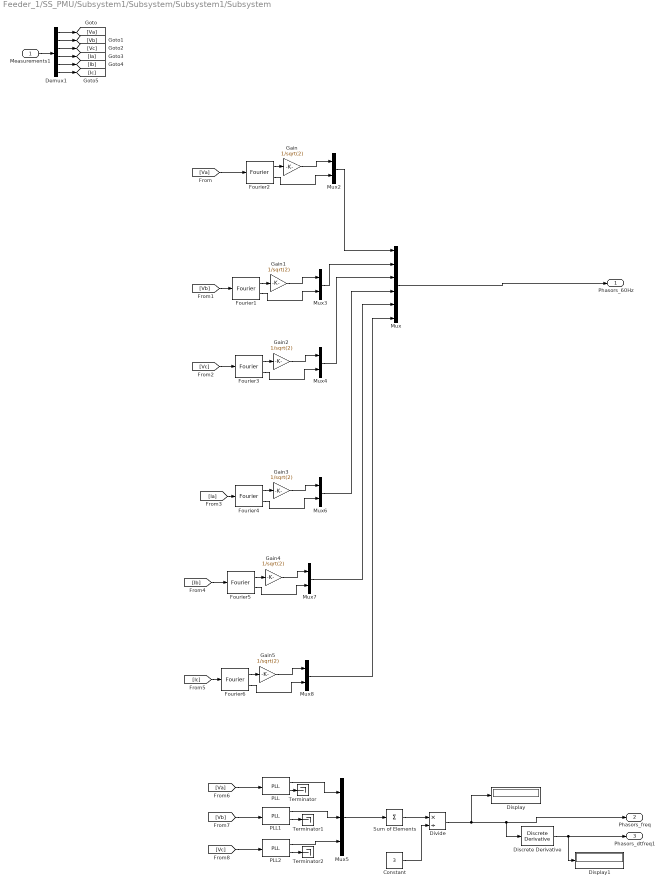
== system Feeder_1/SS_PMU/Subsystem1/Subsystem/Subsystem1/Subsystem ==
  Measurements1 : Inport
  Constant : Constant  Value=3
  Demux1 : Demux  Outputs=6
  Discrete Derivative : simulink/Discrete/Discrete Derivative  gainval=1.0  ICPrevScaledInput=0.0  InputProcessing=Inherited  OutMin=[]  OutMax=[]  OutDataType=fixdt(1, 16)  OutScaling=2^-10  DoSatur=off
  Display : Display
  Display1 : Display
  Divide : Product  Inputs=*/
  Fourier{1..6} (6 alike) : powerlib_meascontrol/Measurements/Fourier  Freq=60  n=1  InInit=[0, 0]  Ts=Ts
  Gain{,1..5} (6 alike) : Gain  Gain=1/sqrt(2)
  Mux : Mux  Inputs=6
  Mux{2..4,6..8} (6 alike) : Mux  Inputs=2
  Mux5 : Mux  Inputs=3
  PLL : powerlib_meascontrol/PLL/PLL  Fmin=60  Par_Init=[0, 60]  ParK=[180, 3200, 1]  TcD=1.6e-4  MaxRateChangeFreq=12  FilterCutOffFreq=25  Ts=Ts  AGC=on
  PLL1 : powerlib_meascontrol/PLL/PLL  Fmin=60  Par_Init=[0, 60]  ParK=[180, 3200, 1]  TcD=1.6e-4  MaxRateChangeFreq=12  FilterCutOffFreq=25  Ts=Ts  AGC=on
  PLL2 : powerlib_meascontrol/PLL/PLL  Fmin=60  Par_Init=[0, 60]  ParK=[180, 3200, 1]  TcD=1.6e-4  MaxRateChangeFreq=12  FilterCutOffFreq=25  Ts=Ts  AGC=on
  Sum of Elements : Sum  Inputs=+
  Terminator : Terminator
  Terminator1 : Terminator
  Terminator2 : Terminator
  Phasors_60Hz : Outport
  Phasors_freq : Outport  Port=2
  Phasors_dtfreq1 : Outport  Port=3
  wires:
  Mux5/1 -> Sum of Elements/1
  PLL2/1 -> Mux5/3
  PLL1/1 -> Mux5/2
  PLL/1 -> Mux5/1
  PLL2/2 -> Terminator2/1
  PLL1/2 -> Terminator1/1
  PLL/2 -> Terminator/1
  [Vc] -> PLL2/1
  [Vb] -> PLL1/1
  [Va] -> PLL/1
  Discrete Derivative/1 -> Display1/1, Phasors_dtfreq1/1
  Mux3/1 -> Mux/2
  Mux2/1 -> Mux/1
  Demux1/2 -> [Vb]
  Measurements1/1 -> Demux1/1
  [Va] -> Fourier2/1
  Demux1/3 -> [Vc]
  Demux1/1 -> [Va]
  Mux7/1 -> Mux/5
  Mux4/1 -> Mux/3
  Mux/1 -> Phasors_60Hz/1
  Demux1/4 -> [Ia]
  Demux1/6 -> [Ic]
  Demux1/5 -> [Ib]
  Mux8/1 -> Mux/6
  Mux6/1 -> Mux/4
  Sum of Elements/1 -> Divide/1
  Divide/1 -> Display/1, Discrete Derivative/1, Phasors_freq/1
  Constant/1 -> Divide/2
  Fourier2/2 -> Mux2/2
  [Vc] -> Fourier3/1
  [Ia] -> Fourier4/1
  Fourier2/1 -> Gain/1
  Gain/1 -> Mux2/1
  [Vb] -> Fourier1/1
  Fourier1/2 -> Mux3/2
  Fourier1/1 -> Gain1/1
  Gain1/1 -> Mux3/1
  Fourier3/2 -> Mux4/2
  Fourier3/1 -> Gain2/1
  Gain2/1 -> Mux4/1
  Fourier4/2 -> Mux6/2
  Fourier4/1 -> Gain3/1
  Gain3/1 -> Mux6/1
  Fourier5/2 -> Mux7/2
  Fourier5/1 -> Gain4/1
  Gain4/1 -> Mux7/1
  Fourier6/2 -> Mux8/2
  Fourier6/1 -> Gain5/1
  Gain5/1 -> Mux8/1
  [Ic] -> Fourier6/1
  [Ib] -> Fourier5/1

== system Feeder_1/SS_PMU/Subsystem10/Subsystem/Subsystem1/Degree to radian1 ==
  Degree : Inport
  Constant : Constant  Value=pi
  Constant1 : Constant  Value=180
  Divide : Product  Inputs=*/
  Product : Product  RndMeth=Zero
  Radian : Outport
  wires:
  Divide/1 -> Radian/1
  Degree/1 -> Product/1
  Constant1/1 -> Divide/2
  Product/1 -> Divide/1
  Constant/1 -> Product/2

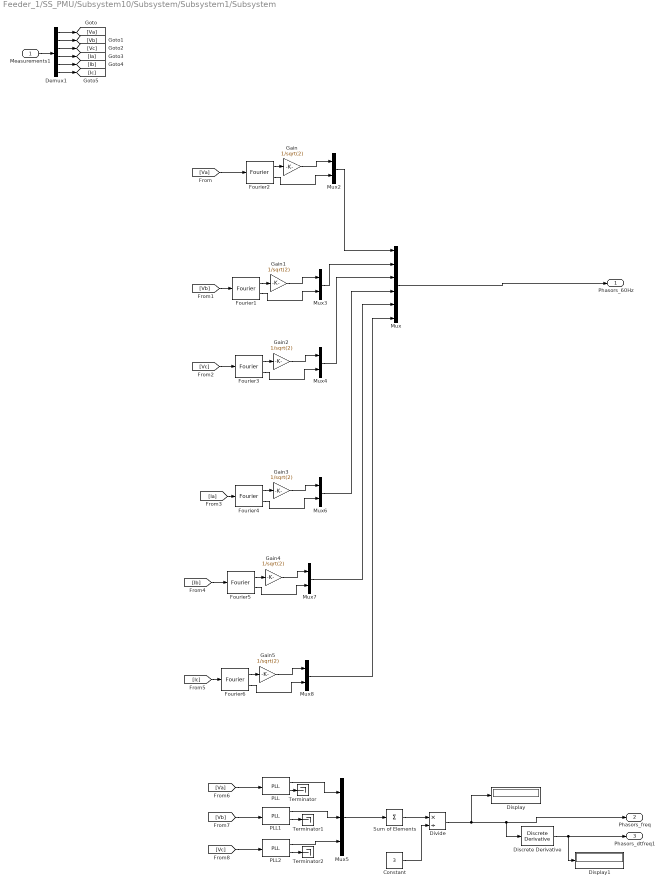
== system Feeder_1/SS_PMU/Subsystem10/Subsystem/Subsystem1/Subsystem ==
  Measurements1 : Inport
  Constant : Constant  Value=3
  Demux1 : Demux  Outputs=6
  Discrete Derivative : simulink/Discrete/Discrete Derivative  gainval=1.0  ICPrevScaledInput=0.0  InputProcessing=Inherited  OutMin=[]  OutMax=[]  OutDataType=fixdt(1, 16)  OutScaling=2^-10  DoSatur=off
  Display : Display
  Display1 : Display
  Divide : Product  Inputs=*/
  Fourier{1..6} (6 alike) : powerlib_meascontrol/Measurements/Fourier  Freq=60  n=1  InInit=[0, 0]  Ts=Ts
  Gain{,1..5} (6 alike) : Gain  Gain=1/sqrt(2)
  Mux : Mux  Inputs=6
  Mux{2..4,6..8} (6 alike) : Mux  Inputs=2
  Mux5 : Mux  Inputs=3
  PLL : powerlib_meascontrol/PLL/PLL  Fmin=60  Par_Init=[0, 60]  ParK=[180, 3200, 1]  TcD=1.6e-4  MaxRateChangeFreq=12  FilterCutOffFreq=25  Ts=Ts  AGC=on
  PLL1 : powerlib_meascontrol/PLL/PLL  Fmin=60  Par_Init=[0, 60]  ParK=[180, 3200, 1]  TcD=1.6e-4  MaxRateChangeFreq=12  FilterCutOffFreq=25  Ts=Ts  AGC=on
  PLL2 : powerlib_meascontrol/PLL/PLL  Fmin=60  Par_Init=[0, 60]  ParK=[180, 3200, 1]  TcD=1.6e-4  MaxRateChangeFreq=12  FilterCutOffFreq=25  Ts=Ts  AGC=on
  Sum of Elements : Sum  Inputs=+
  Terminator : Terminator
  Terminator1 : Terminator
  Terminator2 : Terminator
  Phasors_60Hz : Outport
  Phasors_freq : Outport  Port=2
  Phasors_dtfreq1 : Outport  Port=3
  wires:
  Mux5/1 -> Sum of Elements/1
  PLL2/1 -> Mux5/3
  PLL1/1 -> Mux5/2
  PLL/1 -> Mux5/1
  PLL2/2 -> Terminator2/1
  PLL1/2 -> Terminator1/1
  PLL/2 -> Terminator/1
  [Vc] -> PLL2/1
  [Vb] -> PLL1/1
  [Va] -> PLL/1
  Discrete Derivative/1 -> Display1/1, Phasors_dtfreq1/1
  Mux3/1 -> Mux/2
  Mux2/1 -> Mux/1
  Demux1/2 -> [Vb]
  Measurements1/1 -> Demux1/1
  [Va] -> Fourier2/1
  Demux1/3 -> [Vc]
  Demux1/1 -> [Va]
  Mux7/1 -> Mux/5
  Mux4/1 -> Mux/3
  Mux/1 -> Phasors_60Hz/1
  Demux1/4 -> [Ia]
  Demux1/6 -> [Ic]
  Demux1/5 -> [Ib]
  Mux8/1 -> Mux/6
  Mux6/1 -> Mux/4
  Sum of Elements/1 -> Divide/1
  Divide/1 -> Display/1, Discrete Derivative/1, Phasors_freq/1
  Constant/1 -> Divide/2
  Fourier2/2 -> Mux2/2
  [Vc] -> Fourier3/1
  [Ia] -> Fourier4/1
  Fourier2/1 -> Gain/1
  Gain/1 -> Mux2/1
  [Vb] -> Fourier1/1
  Fourier1/2 -> Mux3/2
  Fourier1/1 -> Gain1/1
  Gain1/1 -> Mux3/1
  Fourier3/2 -> Mux4/2
  Fourier3/1 -> Gain2/1
  Gain2/1 -> Mux4/1
  Fourier4/2 -> Mux6/2
  Fourier4/1 -> Gain3/1
  Gain3/1 -> Mux6/1
  Fourier5/2 -> Mux7/2
  Fourier5/1 -> Gain4/1
  Gain4/1 -> Mux7/1
  Fourier6/2 -> Mux8/2
  Fourier6/1 -> Gain5/1
  Gain5/1 -> Mux8/1
  [Ic] -> Fourier6/1
  [Ib] -> Fourier5/1

== system Feeder_1/SS_PMU/Subsystem11/Subsystem/Subsystem1/Degree to radian1 ==
  Degree : Inport
  Constant : Constant  Value=pi
  Constant1 : Constant  Value=180
  Divide : Product  Inputs=*/
  Product : Product  RndMeth=Zero
  Radian : Outport
  wires:
  Divide/1 -> Radian/1
  Degree/1 -> Product/1
  Constant1/1 -> Divide/2
  Product/1 -> Divide/1
  Constant/1 -> Product/2

== system Feeder_1/SS_PMU/Subsystem11/Subsystem/Subsystem1/Subsystem ==
  Measurements1 : Inport
  Constant : Constant  Value=3
  Constant{1..5} (5 alike) : Constant  Value=0
  Demux1 : Demux  Outputs=2
  Discrete Derivative : simulink/Discrete/Discrete Derivative  gainval=1.0  ICPrevScaledInput=0.0  InputProcessing=Inherited  OutMin=[]  OutMax=[]  OutDataType=fixdt(1, 16)  OutScaling=2^-10  DoSatur=off
  Display : Display
  Display1 : Display
  Divide : Product  Inputs=*/
  Fourier3 : powerlib_meascontrol/Measurements/Fourier  Freq=60  n=1  InInit=[0, 0]  Ts=Ts
  Fourier6 : powerlib_meascontrol/Measurements/Fourier  Freq=60  n=1  InInit=[0, 0]  Ts=Ts
  Gain2 : Gain  Gain=1/sqrt(2)
  Gain5 : Gain  Gain=1/sqrt(2)
  Mux : Mux  Inputs=6
  Mux{2..4,6..8} (6 alike) : Mux  Inputs=2
  Mux5 : Mux  Inputs=3
  PLL2 : powerlib_meascontrol/PLL/PLL  Fmin=60  Par_Init=[0, 60]  ParK=[180, 3200, 1]  TcD=1.6e-4  MaxRateChangeFreq=12  FilterCutOffFreq=25  Ts=Ts  AGC=on
  Sum of Elements : Sum  Inputs=+
  Terminator2 : Terminator
  Phasors_60Hz : Outport
  Phasors_freq : Outport  Port=2
  Phasors_dtfreq1 : Outport  Port=3
  wires:
  Mux5/1 -> Sum of Elements/1
  PLL2/1 -> Mux5/3
  PLL2/2 -> Terminator2/1
  [Vc] -> PLL2/1
  Discrete Derivative/1 -> Display1/1, Phasors_dtfreq1/1
  Mux3/1 -> Mux/2
  Mux2/1 -> Mux/1
  Measurements1/1 -> Demux1/1
  Demux1/1 -> [Vc]
  Mux7/1 -> Mux/5
  Mux4/1 -> Mux/3
  Mux/1 -> Phasors_60Hz/1
  Demux1/2 -> [Ic]
  ? -> ?
  Mux8/1 -> Mux/6
  Mux6/1 -> Mux/4
  Sum of Elements/1 -> Divide/1
  Divide/1 -> Display/1, Discrete Derivative/1, Phasors_freq/1
  Constant/1 -> Divide/2
  [Vc] -> Fourier3/1
  Fourier3/2 -> Mux4/2
  Fourier3/1 -> Gain2/1
  Gain2/1 -> Mux4/1
  Constant2/1 -> Mux7/2, Mux7/1
  Fourier6/2 -> Mux8/2
  Fourier6/1 -> Gain5/1
  Gain5/1 -> Mux8/1
  [Ic] -> Fourier6/1
  Constant1/1 -> Mux5/2, Mux5/1
  Constant3/1 -> Mux6/1, Mux6/2
  Constant4/1 -> Mux2/1, Mux2/2
  Constant5/1 -> Mux3/2, Mux3/1

== system Feeder_1/SS_PMU/Subsystem12/Subsystem/Subsystem1/Degree to radian1 ==
  Degree : Inport
  Constant : Constant  Value=pi
  Constant1 : Constant  Value=180
  Divide : Product  Inputs=*/
  Product : Product  RndMeth=Zero
  Radian : Outport
  wires:
  Divide/1 -> Radian/1
  Degree/1 -> Product/1
  Constant1/1 -> Divide/2
  Product/1 -> Divide/1
  Constant/1 -> Product/2

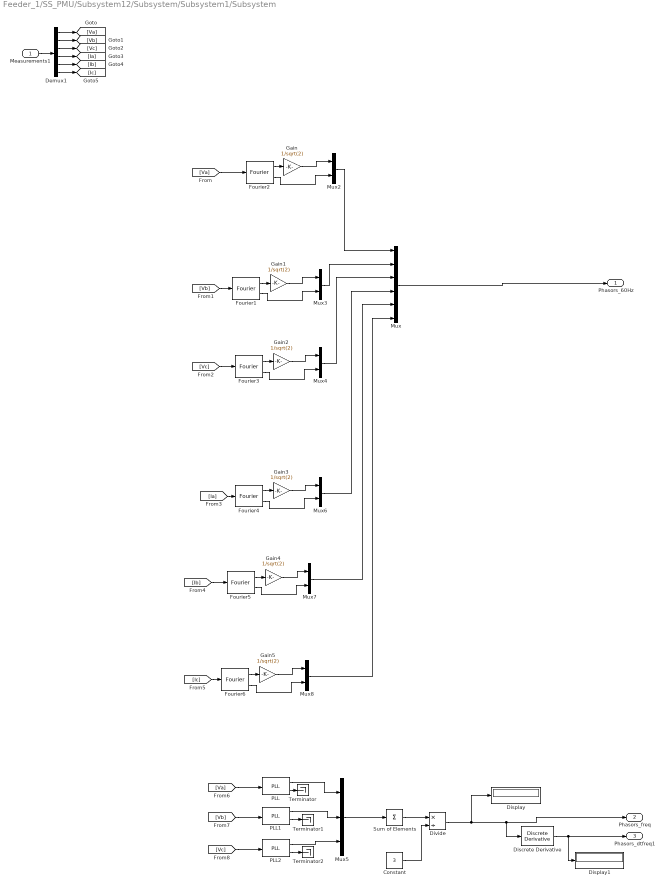
== system Feeder_1/SS_PMU/Subsystem12/Subsystem/Subsystem1/Subsystem ==
  Measurements1 : Inport
  Constant : Constant  Value=3
  Demux1 : Demux  Outputs=6
  Discrete Derivative : simulink/Discrete/Discrete Derivative  gainval=1.0  ICPrevScaledInput=0.0  InputProcessing=Inherited  OutMin=[]  OutMax=[]  OutDataType=fixdt(1, 16)  OutScaling=2^-10  DoSatur=off
  Display : Display
  Display1 : Display
  Divide : Product  Inputs=*/
  Fourier{1..6} (6 alike) : powerlib_meascontrol/Measurements/Fourier  Freq=60  n=1  InInit=[0, 0]  Ts=Ts
  Gain{,1..5} (6 alike) : Gain  Gain=1/sqrt(2)
  Mux : Mux  Inputs=6
  Mux{2..4,6..8} (6 alike) : Mux  Inputs=2
  Mux5 : Mux  Inputs=3
  PLL : powerlib_meascontrol/PLL/PLL  Fmin=60  Par_Init=[0, 60]  ParK=[180, 3200, 1]  TcD=1.6e-4  MaxRateChangeFreq=12  FilterCutOffFreq=25  Ts=Ts  AGC=on
  PLL1 : powerlib_meascontrol/PLL/PLL  Fmin=60  Par_Init=[0, 60]  ParK=[180, 3200, 1]  TcD=1.6e-4  MaxRateChangeFreq=12  FilterCutOffFreq=25  Ts=Ts  AGC=on
  PLL2 : powerlib_meascontrol/PLL/PLL  Fmin=60  Par_Init=[0, 60]  ParK=[180, 3200, 1]  TcD=1.6e-4  MaxRateChangeFreq=12  FilterCutOffFreq=25  Ts=Ts  AGC=on
  Sum of Elements : Sum  Inputs=+
  Terminator : Terminator
  Terminator1 : Terminator
  Terminator2 : Terminator
  Phasors_60Hz : Outport
  Phasors_freq : Outport  Port=2
  Phasors_dtfreq1 : Outport  Port=3
  wires:
  Mux5/1 -> Sum of Elements/1
  PLL2/1 -> Mux5/3
  PLL1/1 -> Mux5/2
  PLL/1 -> Mux5/1
  PLL2/2 -> Terminator2/1
  PLL1/2 -> Terminator1/1
  PLL/2 -> Terminator/1
  [Vc] -> PLL2/1
  [Vb] -> PLL1/1
  [Va] -> PLL/1
  Discrete Derivative/1 -> Display1/1, Phasors_dtfreq1/1
  Mux3/1 -> Mux/2
  Mux2/1 -> Mux/1
  Demux1/2 -> [Vb]
  Measurements1/1 -> Demux1/1
  [Va] -> Fourier2/1
  Demux1/3 -> [Vc]
  Demux1/1 -> [Va]
  Mux7/1 -> Mux/5
  Mux4/1 -> Mux/3
  Mux/1 -> Phasors_60Hz/1
  Demux1/4 -> [Ia]
  Demux1/6 -> [Ic]
  Demux1/5 -> [Ib]
  Mux8/1 -> Mux/6
  Mux6/1 -> Mux/4
  Sum of Elements/1 -> Divide/1
  Divide/1 -> Display/1, Discrete Derivative/1, Phasors_freq/1
  Constant/1 -> Divide/2
  Fourier2/2 -> Mux2/2
  [Vc] -> Fourier3/1
  [Ia] -> Fourier4/1
  Fourier2/1 -> Gain/1
  Gain/1 -> Mux2/1
  [Vb] -> Fourier1/1
  Fourier1/2 -> Mux3/2
  Fourier1/1 -> Gain1/1
  Gain1/1 -> Mux3/1
  Fourier3/2 -> Mux4/2
  Fourier3/1 -> Gain2/1
  Gain2/1 -> Mux4/1
  Fourier4/2 -> Mux6/2
  Fourier4/1 -> Gain3/1
  Gain3/1 -> Mux6/1
  Fourier5/2 -> Mux7/2
  Fourier5/1 -> Gain4/1
  Gain4/1 -> Mux7/1
  Fourier6/2 -> Mux8/2
  Fourier6/1 -> Gain5/1
  Gain5/1 -> Mux8/1
  [Ic] -> Fourier6/1
  [Ib] -> Fourier5/1

== system Feeder_1/SS_PMU/Subsystem13/Subsystem/Subsystem1/Degree to radian1 ==
  Degree : Inport
  Constant : Constant  Value=pi
  Constant1 : Constant  Value=180
  Divide : Product  Inputs=*/
  Product : Product  RndMeth=Zero
  Radian : Outport
  wires:
  Divide/1 -> Radian/1
  Degree/1 -> Product/1
  Constant1/1 -> Divide/2
  Product/1 -> Divide/1
  Constant/1 -> Product/2
